simulink model "JointSpaceControl_own_MCP"  (R2013a)
settings: Solver=ode45  StartTime=0.0  StopTime=sim_end  MaxStep=0.008  RelTol=1e-3
PreLoadFcn:
  | Initialization
InitFcn:
  | Initialization
values from neighbouring files (symbols this model uses):
  a_max = [27 27 27 27 27 27]    [Initialization.m]
  dq_0 = qd_actual.signals.values(1,:)    [Initialization.m]
  K_0 = [            omega_1, zeros(1,5);         0,          omega_2, zeros(1,4);         zeros(1,2), omega_3, zeros(1,3);         zeros(1,3), omega_4, zeros(1,2);         zeros(1,4), omega_5, 0;         zeros(1,5), omega_6]    [Initialization.m]
  K_1 = [            omega_7, zeros(1,5);         0,          omega_8, zeros(1,4);         zeros(1,2), omega_9, zeros(1,3);         zeros(1,3), omega_10, zeros(1,2);         zeros(1,4), omega_11, 0;         zeros(1,5), omega_12]    [Initialization.m]
  q_0 = q_actual.signals.values(1,:)    [Initialization.m]
  q_max = 2*pi*ones(1,6)    [Initialization.m]
  q_min = -2*pi*ones(1,6)    [Initialization.m]
  torque_max = [150 150 150 28 28 28]    [Initialization.m]
  v_max = 3.4*ones(1,6)    [Initialization.m]
(part 3 of 4)

== matlab function JointSpaceControl_own_MCP/Forward & Velocity Kinematics Joint -> Tool Geometric Jacobian/J (made by Michael) ==
  data: J0 output; q input; Tn output
function [J0, Tn] = ur5_jacobian( q )
%UNTITLED J0 returns the jacobian in the inertial frame. Tn returns the
%transformation from origin to end-effector (forward kinematics).

%Defining input ports
q1 = q(1);
q2 = q(2);
q3 = q(3);
q4 = q(4);
q5 = q(5);
q6 = q(6);

% Jacobian (end-effector frame)
Jn1 = [ (35967658190210792782316868215998932771611847913227196662655717226173663198915229*cos(q5 - q6))/106799351796045504119751085308477605730135226117832638497352080391110986289032027501148104346828800 + (84451879200365687*sin(q2 - q6))/6490371073168534535663120411525120 + (194949711497644156173*sin(q4 - q6))/16225927682921336339157801028812800000 - (194949711497644156173*sin(q2 + q3 + q6))/16225927682921336339157801028812800000 + (275840770609662734656058457562955*sin(q2 + q5 + q6))/2596148429267413814265248164610048 - (84451879200365687*sin(q3 + q4 + q6))/6490371073168534535663120411525120 - (2053060087794098037004962814352767697732810782616901170279221510647830364092218317*sin(q4 + q5 + q6))/341757925747345613183203472987128338336432723577064443191526657251555156124902488003673933909852160 - (127350816012176408189502377060506389*sin(q2 + q3 - q5 - q6))/1298074214633706907132624082305024000 - (111172761678833366316347747967194492076366052381217435623730136019215778584537765*sin(q3 + q4 - q5 - q6))/17087896287367280659160173649356416916821636178853222159576332862577757806245124400183696695492608 + (519875567647652786170952659526825091883968323036151981961339556365617307809635277352352397416158688535123641112322663680196253259*cos(q2 + q3 + q4 + q5 - q6))/17329185588255092872365088650894273146477731721098853594815497378841383173785160143999840038150872363108695068508772323931088486400 + (2122825234561248616893610494268290878536612480468246686583653420460184422081415019027164128055730209555068108774478778867800150153*cos(q2 + q3 + q4 - q5 + q6))/86645927941275464361825443254471365732388658605494267974077486894206915868925800719999200190754361815543475342543861619655442432000 + (194949711497644156173*sin(q2 + q3 - q6))/16225927682921336339157801028812800000 + (1379203853048313504376533887083401*sin(q2 + q5 - q6))/12980742146337069071326240823050240 - (1379203853048313504376533887083401*sin(q2 - q5 + q6))/12980742146337069071326240823050240 + (84451879200365687*sin(q3 + q4 - q6))/6490371073168534535663120411525120 - (51326502194852444639440407923254275912386270512895480308024020327083350576388417787*sin(q4 + q5 - q6))/8543948143683640329580086824678208458410818089426611079788166431288878903122562200091848347746304000 - (1283162554871310958843918637192253228892250922824946721836627660932782523731312344957*sin(q4 - q5 + q6))/213598703592091008239502170616955211460270452235665276994704160782221972578064055002296208693657600000 + (191*cos(q2 + q3 + q4 + q6))/2000 + (127350816012176408189502377060506389*sin(q2 + q3 + q5 + q6))/1298074214633706907132624082305024000 - (111172761678833379931084422202676435483582369162931350478896764012094883767702875*sin(q3 + q4 + q5 + q6))/17087896287367280659160173649356416916821636178853222159576332862577757806245124400183696695492608 + (2861063719675858867154458072038785344359566180156884446265273330888120000481209071*cos(q5 + q6))/533996758980227520598755426542388028650676130589163192486760401955554931445160137505740521734144000 - (84451879200365687*sin(q2 + q6))/6490371073168534535663120411525120 - (194949711497644156173*sin(q4 + q6))/16225927682921336339157801028812800000 - (1429657811031045161970119813698793047136231009974723550987905358752535048856873346718200821789284381747153397866676246912996806793*cos(q2 + q3 + q4 - q5 - q6))/86645927941275464361825443254471365732388658605494267974077486894206915868925800719999200190754361815543475342543861619655442432000 - (1011823238475430797566174171647961*cos(q6))/3291009114642412084309938365114701009965471731267159726697218048000 - (275840770609662734656058457562955*sin(q2 - q5 - q6))/2596148429267413814265248164610048 - (51326502194852444639440407923254275912386270512895480308024020327083350576388417787*sin(q4 - q5 - q6))/8543948143683640329580086824678208458410818089426611079788166431288878903122562200091848347746304000 - (27*cos(q2 + q3 + q4 - q6))/2000 + (3183770400304409814838136431224347379*sin(q2 + q3 + q5 - q6))/32451855365842672678315602057625600000 - (3183770400304409814838136431224347379*sin(q2 + q3 - q5 + q6))/32451855365842672678315602057625600000 - (111172761678833366316347747967194492076366052381217435623730136019215778584537765*sin(q3 + q4 + q5 - q6))/17087896287367280659160173649356416916821636178853222159576332862577757806245124400183696695492608 - (555863808394166763508055368658571079967593346278931128385257758985228012726659783*sin(q3 + q4 - q5 + q6))/85439481436836403295800868246782084584108180894266110797881664312888789031225622000918483477463040 + (6151860883830558723075280489357521634050976598849036133515047236737481169606567320141085730345932291258072846594526784421861331081*cos(q2 + q3 + q4 + q5 + q6))/86645927941275464361825443254471365732388658605494267974077486894206915868925800719999200190754361815543475342543861619655442432000, (3772528186279210902532250340080927*cos(q5)*cos(q6))/40564819207303340847894502572032000 - (203678061600881951*cos(q6))/40564819207303340847894502572032000 - (39243*cos(q4)*sin(q6))/100000 - (269862747400677809654420514623322019689666659727888053949852700633*sin(q5)*sin(q6))/3291009114642412084309938365114701009965471731267159726697218048000 + (17*sin(q3)*sin(q4)*sin(q6))/40 + (194949711497644156173*sin(q4)*sin(q5)*sin(q6))/8112963841460668169578900514406400000 - (17*cos(q3)*cos(q4)*sin(q6))/40 - (968462910914422702168033488243437403*cos(q4)*cos(q5)*sin(q6))/658201822928482416861987673022940201993094346253431945339443609600000 - (194949711497644156173*cos(q4)*cos(q6)*sin(q5))/8112963841460668169578900514406400000 - (39243*cos(q5)*cos(q6)*sin(q4))/100000 - (419536464733715208746950266293057*cos(q3)*cos(q4)*cos(q5)*sin(q6))/263280729171392966744795069209176080797237738501372778135777443840 - (84451879200365687*cos(q3)*cos(q4)*cos(q6)*sin(q5))/3245185536584267267831560205762560 - (17*cos(q3)*cos(q5)*cos(q6)*sin(q4))/40 - (17*cos(q4)*cos(q5)*cos(q6)*sin(q3))/40 + (84451879200365687*cos(q3)*sin(q4)*sin(q5)*sin(q6))/3245185536584267267831560205762560 + (84451879200365687*cos(q4)*sin(q3)*sin(q5)*sin(q6))/3245185536584267267831560205762560 + (419536464733715208746950266293057*cos(q5)*sin(q3)*sin(q4)*sin(q6))/263280729171392966744795069209176080797237738501372778135777443840 + (84451879200365687*cos(q6)*sin(q3)*sin(q4)*sin(q5))/3245185536584267267831560205762560, (3772528186279210902532250340080927*cos(q5)*cos(q6))/40564819207303340847894502572032000 - (203678061600881951*cos(q6))/40564819207303340847894502572032000 - (39243*cos(q4)*sin(q6))/100000 - (269862747400677809654420514623322019689666659727888053949852700633*sin(q5)*sin(q6))/3291009114642412084309938365114701009965471731267159726697218048000 + (194949711497644156173*sin(q4)*sin(q5)*sin(q6))/8112963841460668169578900514406400000 - (968462910914422702168033488243437403*cos(q4)*cos(q5)*sin(q6))/658201822928482416861987673022940201993094346253431945339443609600000 - (194949711497644156173*cos(q4)*cos(q6)*sin(q5))/8112963841460668169578900514406400000 - (39243*cos(q5)*cos(q6)*sin(q4))/100000, (3772528186279210902532250340080927*cos(q5)*cos(q6))/40564819207303340847894502572032000 - (203678061600881951*cos(q6))/40564819207303340847894502572032000 - (269862747400677809654420514623322019689666659727888053949852700633*sin(q5)*sin(q6))/3291009114642412084309938365114701009965471731267159726697218048000,                                 -(41*cos(q6))/500, 0];
Jn2 = [ (35967658190210792782316868215998932771611847913227196662655717226173663198915229*sin(q5 - q6))/106799351796045504119751085308477605730135226117832638497352080391110986289032027501148104346828800 - (194949711497644156173*cos(q4 - q6))/16225927682921336339157801028812800000 - (6151860883830558723075280489357521634050976598849036133515047236737481169606567320141085730345932291258072846594526784421861331081*sin(q2 + q3 + q4 + q5 + q6))/86645927941275464361825443254471365732388658605494267974077486894206915868925800719999200190754361815543475342543861619655442432000 - (84451879200365687*cos(q2 - q6))/6490371073168534535663120411525120 - (194949711497644156173*cos(q2 + q3 + q6))/16225927682921336339157801028812800000 + (275840770609662734656058457562955*cos(q2 + q5 + q6))/2596148429267413814265248164610048 - (84451879200365687*cos(q3 + q4 + q6))/6490371073168534535663120411525120 - (2053060087794098037004962814352767697732810782616901170279221510647830364092218317*cos(q4 + q5 + q6))/341757925747345613183203472987128338336432723577064443191526657251555156124902488003673933909852160 + (127350816012176408189502377060506389*cos(q2 + q3 - q5 - q6))/1298074214633706907132624082305024000 + (111172761678833366316347747967194492076366052381217435623730136019215778584537765*cos(q3 + q4 - q5 - q6))/17087896287367280659160173649356416916821636178853222159576332862577757806245124400183696695492608 + (519875567647652786170952659526825091883968323036151981961339556365617307809635277352352397416158688535123641112322663680196253259*sin(q2 + q3 + q4 + q5 - q6))/17329185588255092872365088650894273146477731721098853594815497378841383173785160143999840038150872363108695068508772323931088486400 - (2122825234561248616893610494268290878536612480468246686583653420460184422081415019027164128055730209555068108774478778867800150153*sin(q2 + q3 + q4 - q5 + q6))/86645927941275464361825443254471365732388658605494267974077486894206915868925800719999200190754361815543475342543861619655442432000 - (194949711497644156173*cos(q2 + q3 - q6))/16225927682921336339157801028812800000 - (1379203853048313504376533887083401*cos(q2 + q5 - q6))/12980742146337069071326240823050240 - (1379203853048313504376533887083401*cos(q2 - q5 + q6))/12980742146337069071326240823050240 - (84451879200365687*cos(q3 + q4 - q6))/6490371073168534535663120411525120 + (51326502194852444639440407923254275912386270512895480308024020327083350576388417787*cos(q4 + q5 - q6))/8543948143683640329580086824678208458410818089426611079788166431288878903122562200091848347746304000 - (1283162554871310958843918637192253228892250922824946721836627660932782523731312344957*cos(q4 - q5 + q6))/213598703592091008239502170616955211460270452235665276994704160782221972578064055002296208693657600000 + (127350816012176408189502377060506389*cos(q2 + q3 + q5 + q6))/1298074214633706907132624082305024000 - (111172761678833379931084422202676435483582369162931350478896764012094883767702875*cos(q3 + q4 + q5 + q6))/17087896287367280659160173649356416916821636178853222159576332862577757806245124400183696695492608 - (191*sin(q2 + q3 + q4 + q6))/2000 - (84451879200365687*cos(q2 + q6))/6490371073168534535663120411525120 - (194949711497644156173*cos(q4 + q6))/16225927682921336339157801028812800000 - (2861063719675858867154458072038785344359566180156884446265273330888120000481209071*sin(q5 + q6))/533996758980227520598755426542388028650676130589163192486760401955554931445160137505740521734144000 - (1429657811031045161970119813698793047136231009974723550987905358752535048856873346718200821789284381747153397866676246912996806793*sin(q2 + q3 + q4 - q5 - q6))/86645927941275464361825443254471365732388658605494267974077486894206915868925800719999200190754361815543475342543861619655442432000 + (275840770609662734656058457562955*cos(q2 - q5 - q6))/2596148429267413814265248164610048 + (51326502194852444639440407923254275912386270512895480308024020327083350576388417787*cos(q4 - q5 - q6))/8543948143683640329580086824678208458410818089426611079788166431288878903122562200091848347746304000 + (1011823238475430797566174171647961*sin(q6))/3291009114642412084309938365114701009965471731267159726697218048000 - (3183770400304409814838136431224347379*cos(q2 + q3 + q5 - q6))/32451855365842672678315602057625600000 - (3183770400304409814838136431224347379*cos(q2 + q3 - q5 + q6))/32451855365842672678315602057625600000 + (111172761678833366316347747967194492076366052381217435623730136019215778584537765*cos(q3 + q4 + q5 - q6))/17087896287367280659160173649356416916821636178853222159576332862577757806245124400183696695492608 - (555863808394166763508055368658571079967593346278931128385257758985228012726659783*cos(q3 + q4 - q5 + q6))/85439481436836403295800868246782084584108180894266110797881664312888789031225622000918483477463040 - (27*sin(q2 + q3 + q4 - q6))/2000, (203678061600881951*sin(q6))/40564819207303340847894502572032000 - (39243*cos(q4)*cos(q6))/100000 - (3772528186279210902532250340080927*cos(q5)*sin(q6))/40564819207303340847894502572032000 - (269862747400677809654420514623322019689666659727888053949852700633*cos(q6)*sin(q5))/3291009114642412084309938365114701009965471731267159726697218048000 - (17*cos(q3)*cos(q4)*cos(q6))/40 - (968462910914422702168033488243437403*cos(q4)*cos(q5)*cos(q6))/658201822928482416861987673022940201993094346253431945339443609600000 + (17*cos(q6)*sin(q3)*sin(q4))/40 + (194949711497644156173*cos(q4)*sin(q5)*sin(q6))/8112963841460668169578900514406400000 + (39243*cos(q5)*sin(q4)*sin(q6))/100000 + (194949711497644156173*cos(q6)*sin(q4)*sin(q5))/8112963841460668169578900514406400000 - (419536464733715208746950266293057*cos(q3)*cos(q4)*cos(q5)*cos(q6))/263280729171392966744795069209176080797237738501372778135777443840 + (84451879200365687*cos(q3)*cos(q4)*sin(q5)*sin(q6))/3245185536584267267831560205762560 + (17*cos(q3)*cos(q5)*sin(q4)*sin(q6))/40 + (84451879200365687*cos(q3)*cos(q6)*sin(q4)*sin(q5))/3245185536584267267831560205762560 + (17*cos(q4)*cos(q5)*sin(q3)*sin(q6))/40 + (84451879200365687*cos(q4)*cos(q6)*sin(q3)*sin(q5))/3245185536584267267831560205762560 + (419536464733715208746950266293057*cos(q5)*cos(q6)*sin(q3)*sin(q4))/263280729171392966744795069209176080797237738501372778135777443840 - (84451879200365687*sin(q3)*sin(q4)*sin(q5)*sin(q6))/3245185536584267267831560205762560, (203678061600881951*sin(q6))/40564819207303340847894502572032000 - (39243*cos(q4)*cos(q6))/100000 - (3772528186279210902532250340080927*cos(q5)*sin(q6))/40564819207303340847894502572032000 - (269862747400677809654420514623322019689666659727888053949852700633*cos(q6)*sin(q5))/3291009114642412084309938365114701009965471731267159726697218048000 - (968462910914422702168033488243437403*cos(q4)*cos(q5)*cos(q6))/658201822928482416861987673022940201993094346253431945339443609600000 + (194949711497644156173*cos(q4)*sin(q5)*sin(q6))/8112963841460668169578900514406400000 + (39243*cos(q5)*sin(q4)*sin(q6))/100000 + (194949711497644156173*cos(q6)*sin(q4)*sin(q5))/8112963841460668169578900514406400000, (203678061600881951*sin(q6))/40564819207303340847894502572032000 - (3772528186279210902532250340080927*cos(q5)*sin(q6))/40564819207303340847894502572032000 - (269862747400677809654420514623322019689666659727888053949852700633*cos(q6)*sin(q5))/3291009114642412084309938365114701009965471731267159726697218048000,                                  (41*sin(q6))/500, 0];
Jn3 = [                                                                                                                                                                                                                                                                                                                                                                                                                                                                                                                                                                                                                                                                                                                                                                                                                                                                                                                                                                                                                                                                                                                                                                                                                                                                                                                                                                                                                                                                                                                                                                                                                                                                                                                                                                                                                                                                                                                                                                                                                                                                                                                                                                                                                                                                                                                                                                                                                                                                                                                                                                                                                                                                                                                                                                                                                                                                                                                                                                                                                                                                                                                                                                                                                                                                                                                               (17*cos(q2 - q5))/80 + (15816199602835760256257693185578612149839397336469669*cos(q4 - q5))/1316403645856964833723975346045880403986188692506863890678887219200000 + (39243*cos(q2 + q3 + q5))/200000 - (1370310084591942294341002243687833653188636725005*cos(q3 + q4 + q5))/105312291668557186697918027683670432318895095400549111254310977536 + (541485578402344699*sin(q2 + q3 + q4))/81129638414606681695789005144064000 + (39243*cos(q2 + q3 - q5))/200000 + (6851550422959710632632081751008750772042651038911*cos(q3 + q4 - q5))/526561458342785933489590138418352161594475477002745556271554887680 - (1329567682315534563473755419380555181845910000005711135641209403853*sin(q2 + q3 + q4 + q5))/13164036458569648337239753460458804039861886925068638906788872192000 + (968462910914422702168033488243437403*cos(q2 + q3))/658201822928482416861987673022940201993094346253431945339443609600000 + (17*cos(q2 + q5))/80 + (419536464733715208746950266293057*cos(q3 + q4))/263280729171392966744795069209176080797237738501372778135777443840 - (632647984113430487727340600576960659436254952933779*cos(q4 + q5))/52656145834278593348959013841835216159447547700274555627155488768000 + (419536464733715208746950266293057*cos(q2))/263280729171392966744795069209176080797237738501372778135777443840 + (968462910914422702168033488243437403*cos(q4))/658201822928482416861987673022940201993094346253431945339443609600000 - (462001456802000523*sin(q5))/81129638414606681695789005144064000 + (105312291668557180249399982545116558696073684159504065944814356019*sin(q2 + q3 + q4 - q5))/13164036458569648337239753460458804039861886925068638906788872192000,                                                                                                                                                                                                                                                                                                                                                                                                                                                                                                                                                                                                                                                                                                                                                                                                                                                                                                                                                                                       (3183770400304409814838136431224347379*cos(q4 - q5))/16225927682921336339157801028812800000 - (275840770609662734656058457562955*cos(q3 + q4 + q5))/1298074214633706907132624082305024 + (1379203853048313504376533887083401*cos(q3 + q4 - q5))/6490371073168534535663120411525120 + (84451879200365687*cos(q3 + q4))/3245185536584267267831560205762560 - (127350816012176408189502377060506389*cos(q4 + q5))/649037107316853453566312041152512000 + (194949711497644156173*cos(q4))/8112963841460668169578900514406400000 - (93*sin(q5))/1000,                                                                                                                                                                                                                                                                                                                                                                                                                                                                                                              (194949711497644156173*cos(q4))/8112963841460668169578900514406400000 - (93*sin(q5))/1000 - (194949711497644156173*cos(q4)*cos(q5))/8112963841460668169578900514406400000 + (39243*sin(q4)*sin(q5))/100000,                                                                                                                                                                                                                                                                                                     -(93*sin(q5))/1000,                                                 0, 0];
Jn4 = [                                                                                                                                                                                                                                                                                                                                                                                                                                                                                                                                                                                                                                                                                                                                                                                                                                                                                                                                                                                                                                                                                                                                                                                                                                                                                                                                                                                                                                                                                                                                                                                                                                                                                                                                                                                                                                                                                                                                                                                                                                                                                                                                                                                                                                                                                                                                                                                                                                                                                                                                                                                                                                                                                                                                                                                                                                                                                                                                                                                                                                                                                                                                                                                                                                                                                                                                                                                                                                                                                                                                                                                                                                                                                                                                                                                                                                                                                          (6582018229284824974684632372548374012493161295659483273165080625*sin(q2 + q3 + q4 + q5 + q6))/26328072917139296674479506920917608079723773850137277813577744384 + (403032377821159448978357750059338280708391237583*sin(q5 - q6))/13164036458569648337239753460458804039861886925068638906788872192 + (6582018229284824168619876730229377341315370891051451985731712975*sin(q2 + q3 + q4 + q5 - q6))/26328072917139296674479506920917608079723773850137277813577744384 + (6582018229284823362555121087910479384599870772374890568949237809*sin(q2 + q3 + q4 - q5 + q6))/26328072917139296674479506920917608079723773850137277813577744384 + sin(q2 + q3 + q4 + q6)/2 + (403032377821159498335588895202304015643716683825*sin(q5 + q6))/13164036458569648337239753460458804039861886925068638906788872192 + (6582018229284824168619876730229377341315370891051451985731712975*sin(q2 + q3 + q4 - q5 - q6))/26328072917139296674479506920917608079723773850137277813577744384 - (24678615572571482867467662723121*sin(q6))/6582018229284824168619876730229402019930943462534319453394436096 - sin(q2 + q3 + q4 - q6)/2,                                                                                                                                                                                                                                                                                                                                                                                                                                                                                                                                                                                                                                                                                                                                                                                                                                                                                                                                                                                                                                                                                                                                                                                                                                                                                                                                                                                                                             sin(q5) - (4967757600021511*sin(q5/2)^2*sin(q6))/40564819207303340847894502572032 - 2*sin(q6/2)^2*sin(q5),                                                                                                                                                                                                                                                                                                                                                                                                                                                                                                                                                                                                               sin(q5) - (4967757600021511*sin(q5/2)^2*sin(q6))/40564819207303340847894502572032 - 2*sin(q6/2)^2*sin(q5),                                                                                                                                                                                                              sin(q5) - (4967757600021511*sin(q5/2)^2*sin(q6))/40564819207303340847894502572032 - 2*sin(q6/2)^2*sin(q5),                                          -sin(q6), 0];
Jn5 = [                                                                                                                                                                                                                                                                                                                                                                                                                                                                                                                                                                                                                                                                                                                                                                                                                                                                                                                                                                                                                                                                                                                                                                                                                                                                                                                                                                                                                                                                                                                                                                                                                                                                                                                                                                                                                                                                                                                                                                                                                                                                                                                                                                                                                                                                                                                                                                                                                                                                                                                                                                                                                                                                                                                                                                                                                                                                                                                                                                                                                                                                                                                                                                                                                                                                                                                                                                                                                                                                                                                                                                                                                                                                                                                                                                                                                                                                                          (6582018229284823362555121087910479384599870772374890568949237809*cos(q2 + q3 + q4 - q5 + q6))/26328072917139296674479506920917608079723773850137277813577744384 - (6582018229284824168619876730229377341315370891051451985731712975*cos(q2 + q3 + q4 + q5 - q6))/26328072917139296674479506920917608079723773850137277813577744384 - (403032377821159448978357750059338280708391237583*cos(q5 - q6))/13164036458569648337239753460458804039861886925068638906788872192 + cos(q2 + q3 + q4 + q6)/2 + (403032377821159498335588895202304015643716683825*cos(q5 + q6))/13164036458569648337239753460458804039861886925068638906788872192 - (6582018229284824168619876730229377341315370891051451985731712975*cos(q2 + q3 + q4 - q5 - q6))/26328072917139296674479506920917608079723773850137277813577744384 - (24678615572571482867467662723121*cos(q6))/6582018229284824168619876730229402019930943462534319453394436096 + cos(q2 + q3 + q4 - q6)/2 + (6582018229284824974684632372548374012493161295659483273165080625*cos(q2 + q3 + q4 + q5 + q6))/26328072917139296674479506920917608079723773850137277813577744384,                                                                                                                                                                                                                                                                                                                                                                                                                                                                                                                                                                                                                                                                                                                                                                                                                                                                                                                                                                                                                                                                                                                                                                                                                                                                                                                                                                                   (4967757600021511*cos(q5)*cos(q6))/81129638414606681695789005144064 - (4967757600021511*cos(q6))/81129638414606681695789005144064 - sin(q5)*sin(q6),                                                                                                                                                                                                                                                                                                                                                                                                                                                                                                                                                                     (4967757600021511*cos(q5)*cos(q6))/81129638414606681695789005144064 - (4967757600021511*cos(q6))/81129638414606681695789005144064 - sin(q5)*sin(q6),                                                                                                                                                                    (4967757600021511*cos(q5)*cos(q6))/81129638414606681695789005144064 - (4967757600021511*cos(q6))/81129638414606681695789005144064 - sin(q5)*sin(q6),                                          -cos(q6), 0];
Jn6 = [                                                                                                                                                                                                                                                                                                                                                                                                                                                                                                                                                                                                                                                                                                                                                                                                                                                                                                                                                                                                                                                                                                                                                                                                                                                                                                                                                                                                                                                                                                                                                                                                                                                                                                                                                                                                                                                                                                                                                                                                                                                                                                                                                                                                                                                                                                                                                                                                                                                                                                                                                                                                                                                                                                                                                                                                                                                                                                                                                                                                                                                                                                                                                                                                                                                                                                                                                                                                                                                                                                                                                                                                                                                                                                                                                                                                                                                                                                                                                                                                                                                                                                                                                                                                                                                                                                                                                                                                                                                                                                                            (81129638414606686663546605165575*cos(q2 + q3 + q4 + q5))/162259276829213363391578010288128 - (4967757600021511*cos(q2 + q3 + q4))/81129638414606681695789005144064 + (4967757600021511*cos(q5))/81129638414606681695789005144064 - (81129638414606676728031405122553*cos(q2 + q3 + q4 - q5))/162259276829213363391578010288128 + 122597380068651197257713859414983140362437055831/533996758980227520598755426542388028650676130589163192486760401955554931445160137505740521734144,                                                                                                                                                                                                                                                                                                                                                                                                                                                                                                                                                                                                                                                                                                                                                                                                                                                                                                                                                                                                                                                                                                                                                                                                                                                                                                                                                                                                                           cos(q5) + 24678615572571482867467662723121/6582018229284824168619876730229402019930943462534319453394436096,                                                                                                                                                                                                                                                                                                                                                                                                                                                                                                                                                                                                             cos(q5) + 24678615572571482867467662723121/6582018229284824168619876730229402019930943462534319453394436096,                                                                                                                                                                                                            cos(q5) + 24678615572571482867467662723121/6582018229284824168619876730229402019930943462534319453394436096, 4967757600021511/81129638414606681695789005144064, 1];

% Forward kinematics
Tn1 = [   cos(q6)*(sin(q5)*(sin(q1) - (4967757600021511*cos(q4)*(sin(q3)*(cos(q1)*cos(q2) - (4967757600021511*sin(q1)*sin(q2))/81129638414606681695789005144064) + cos(q3)*(cos(q1)*sin(q2) + (4967757600021511*cos(q2)*sin(q1))/81129638414606681695789005144064)))/81129638414606681695789005144064 + (4967757600021511*sin(q4)*(sin(q3)*(cos(q1)*sin(q2) + (4967757600021511*cos(q2)*sin(q1))/81129638414606681695789005144064) - cos(q3)*(cos(q1)*cos(q2) - (4967757600021511*sin(q1)*sin(q2))/81129638414606681695789005144064)))/81129638414606681695789005144064) - cos(q5)*(cos(q4)*(sin(q3)*(cos(q1)*sin(q2) + (4967757600021511*cos(q2)*sin(q1))/81129638414606681695789005144064) - cos(q3)*(cos(q1)*cos(q2) - (4967757600021511*sin(q1)*sin(q2))/81129638414606681695789005144064)) + sin(q4)*(sin(q3)*(cos(q1)*cos(q2) - (4967757600021511*sin(q1)*sin(q2))/81129638414606681695789005144064) + cos(q3)*(cos(q1)*sin(q2) + (4967757600021511*cos(q2)*sin(q1))/81129638414606681695789005144064)))) + sin(q6)*((4967757600021511*cos(q5)*(sin(q1) - (4967757600021511*cos(q4)*(sin(q3)*(cos(q1)*cos(q2) - (4967757600021511*sin(q1)*sin(q2))/81129638414606681695789005144064) + cos(q3)*(cos(q1)*sin(q2) + (4967757600021511*cos(q2)*sin(q1))/81129638414606681695789005144064)))/81129638414606681695789005144064 + (4967757600021511*sin(q4)*(sin(q3)*(cos(q1)*sin(q2) + (4967757600021511*cos(q2)*sin(q1))/81129638414606681695789005144064) - cos(q3)*(cos(q1)*cos(q2) - (4967757600021511*sin(q1)*sin(q2))/81129638414606681695789005144064)))/81129638414606681695789005144064))/81129638414606681695789005144064 - (4967757600021511*sin(q1))/81129638414606681695789005144064 - cos(q4)*(sin(q3)*(cos(q1)*cos(q2) - (4967757600021511*sin(q1)*sin(q2))/81129638414606681695789005144064) + cos(q3)*(cos(q1)*sin(q2) + (4967757600021511*cos(q2)*sin(q1))/81129638414606681695789005144064)) + sin(q4)*(sin(q3)*(cos(q1)*sin(q2) + (4967757600021511*cos(q2)*sin(q1))/81129638414606681695789005144064) - cos(q3)*(cos(q1)*cos(q2) - (4967757600021511*sin(q1)*sin(q2))/81129638414606681695789005144064)) + (4967757600021511*sin(q5)*(cos(q4)*(sin(q3)*(cos(q1)*sin(q2) + (4967757600021511*cos(q2)*sin(q1))/81129638414606681695789005144064) - cos(q3)*(cos(q1)*cos(q2) - (4967757600021511*sin(q1)*sin(q2))/81129638414606681695789005144064)) + sin(q4)*(sin(q3)*(cos(q1)*cos(q2) - (4967757600021511*sin(q1)*sin(q2))/81129638414606681695789005144064) + cos(q3)*(cos(q1)*sin(q2) + (4967757600021511*cos(q2)*sin(q1))/81129638414606681695789005144064))))/81129638414606681695789005144064), cos(q6)*((4967757600021511*cos(q5)*(sin(q1) - (4967757600021511*cos(q4)*(sin(q3)*(cos(q1)*cos(q2) - (4967757600021511*sin(q1)*sin(q2))/81129638414606681695789005144064) + cos(q3)*(cos(q1)*sin(q2) + (4967757600021511*cos(q2)*sin(q1))/81129638414606681695789005144064)))/81129638414606681695789005144064 + (4967757600021511*sin(q4)*(sin(q3)*(cos(q1)*sin(q2) + (4967757600021511*cos(q2)*sin(q1))/81129638414606681695789005144064) - cos(q3)*(cos(q1)*cos(q2) - (4967757600021511*sin(q1)*sin(q2))/81129638414606681695789005144064)))/81129638414606681695789005144064))/81129638414606681695789005144064 - (4967757600021511*sin(q1))/81129638414606681695789005144064 - cos(q4)*(sin(q3)*(cos(q1)*cos(q2) - (4967757600021511*sin(q1)*sin(q2))/81129638414606681695789005144064) + cos(q3)*(cos(q1)*sin(q2) + (4967757600021511*cos(q2)*sin(q1))/81129638414606681695789005144064)) + sin(q4)*(sin(q3)*(cos(q1)*sin(q2) + (4967757600021511*cos(q2)*sin(q1))/81129638414606681695789005144064) - cos(q3)*(cos(q1)*cos(q2) - (4967757600021511*sin(q1)*sin(q2))/81129638414606681695789005144064)) + (4967757600021511*sin(q5)*(cos(q4)*(sin(q3)*(cos(q1)*sin(q2) + (4967757600021511*cos(q2)*sin(q1))/81129638414606681695789005144064) - cos(q3)*(cos(q1)*cos(q2) - (4967757600021511*sin(q1)*sin(q2))/81129638414606681695789005144064)) + sin(q4)*(sin(q3)*(cos(q1)*cos(q2) - (4967757600021511*sin(q1)*sin(q2))/81129638414606681695789005144064) + cos(q3)*(cos(q1)*sin(q2) + (4967757600021511*cos(q2)*sin(q1))/81129638414606681695789005144064))))/81129638414606681695789005144064) - sin(q6)*(sin(q5)*(sin(q1) - (4967757600021511*cos(q4)*(sin(q3)*(cos(q1)*cos(q2) - (4967757600021511*sin(q1)*sin(q2))/81129638414606681695789005144064) + cos(q3)*(cos(q1)*sin(q2) + (4967757600021511*cos(q2)*sin(q1))/81129638414606681695789005144064)))/81129638414606681695789005144064 + (4967757600021511*sin(q4)*(sin(q3)*(cos(q1)*sin(q2) + (4967757600021511*cos(q2)*sin(q1))/81129638414606681695789005144064) - cos(q3)*(cos(q1)*cos(q2) - (4967757600021511*sin(q1)*sin(q2))/81129638414606681695789005144064)))/81129638414606681695789005144064) - cos(q5)*(cos(q4)*(sin(q3)*(cos(q1)*sin(q2) + (4967757600021511*cos(q2)*sin(q1))/81129638414606681695789005144064) - cos(q3)*(cos(q1)*cos(q2) - (4967757600021511*sin(q1)*sin(q2))/81129638414606681695789005144064)) + sin(q4)*(sin(q3)*(cos(q1)*cos(q2) - (4967757600021511*sin(q1)*sin(q2))/81129638414606681695789005144064) + cos(q3)*(cos(q1)*sin(q2) + (4967757600021511*cos(q2)*sin(q1))/81129638414606681695789005144064)))), sin(q1 - q5)/2 - (6582018229284824974684632372548374012493161295659483273165080625*sin(q1 + q2 + q3 + q4 + q5))/26328072917139296674479506920917608079723773850137277813577744384 - (6582018229284823362555121087910479384599870772374890568949237809*sin(q1 - q2 - q3 - q4 + q5))/26328072917139296674479506920917608079723773850137277813577744384 + (6582018229284824168619876730229377341315370891051451985731712975*sin(q1 + q2 + q3 + q4 - q5))/26328072917139296674479506920917608079723773850137277813577744384 + (6582018229284824168619876730229377341315370891051451985731712975*sin(q1 - q2 - q3 - q4 - q5))/26328072917139296674479506920917608079723773850137277813577744384 + (403032377821159498335588895202304015643716683825*sin(q1 + q2 + q3 + q4))/13164036458569648337239753460458804039861886925068638906788872192 + sin(q1 + q5)/2 - (403032377821159448978357750059338280708391237583*sin(q1 - q2 - q3 - q4))/13164036458569648337239753460458804039861886925068638906788872192 + (24678615572571482867467662723121*sin(q1))/6582018229284824168619876730229402019930943462534319453394436096, (41*sin(q1 - q5))/1000 - (2158901979205422591696559418195866676097756904976310513598146445*sin(q1 + q2 + q3 + q4 + q5))/105312291668557186697918027683670432318895095400549111254310977536 - (1379203853048313504376533887083401*cos(q1 - q2))/6490371073168534535663120411525120 - (127350816012176408189502377060506389*cos(q1 + q2 + q3))/649037107316853453566312041152512000 - (269862747400677757864759964604329654768594701667370513326918750169*sin(q1 - q2 - q3 - q4 + q5))/13164036458569648337239753460458804039861886925068638906788872192000 + (10794509896027111636536597837576178839757208261324381256600009279*sin(q1 + q2 + q3 + q4 - q5))/526561458342785933489590138418352161594475477002745556271554887680 + (10794509896027111636536597837576178839757208261324381256600009279*sin(q1 - q2 - q3 - q4 - q5))/526561458342785933489590138418352161594475477002745556271554887680 + (12242553906469774364246293092284886029407723065419755446469379521*sin(q1 + q2 + q3 + q4))/263280729171392966744795069209176080797237738501372778135777443840 - (275840770609662734656058457562955*cos(q1 + q2))/1298074214633706907132624082305024 + (41*sin(q1 + q5))/1000 - (306063847661744321624146189939289076990197121107531973440372846631*sin(q1 - q2 - q3 - q4))/6582018229284824168619876730229402019930943462534319453394436096000 - (3183770400304409814838136431224347379*cos(q1 - q2 - q3))/16225927682921336339157801028812800000 + (358719993496022935930788850481418946958734396472101366570677587929*sin(q1))/3291009114642412084309938365114701009965471731267159726697218048000];
Tn2 = [ - cos(q6)*(sin(q5)*(cos(q1) + (4967757600021511*cos(q4)*(sin(q3)*((4967757600021511*cos(q1)*sin(q2))/81129638414606681695789005144064 + cos(q2)*sin(q1)) - cos(q3)*((4967757600021511*cos(q1)*cos(q2))/81129638414606681695789005144064 - sin(q1)*sin(q2))))/81129638414606681695789005144064 + (4967757600021511*sin(q4)*(sin(q3)*((4967757600021511*cos(q1)*cos(q2))/81129638414606681695789005144064 - sin(q1)*sin(q2)) + cos(q3)*((4967757600021511*cos(q1)*sin(q2))/81129638414606681695789005144064 + cos(q2)*sin(q1))))/81129638414606681695789005144064) - cos(q5)*(cos(q4)*(sin(q3)*((4967757600021511*cos(q1)*cos(q2))/81129638414606681695789005144064 - sin(q1)*sin(q2)) + cos(q3)*((4967757600021511*cos(q1)*sin(q2))/81129638414606681695789005144064 + cos(q2)*sin(q1))) - sin(q4)*(sin(q3)*((4967757600021511*cos(q1)*sin(q2))/81129638414606681695789005144064 + cos(q2)*sin(q1)) - cos(q3)*((4967757600021511*cos(q1)*cos(q2))/81129638414606681695789005144064 - sin(q1)*sin(q2))))) - sin(q6)*((4967757600021511*cos(q5)*(cos(q1) + (4967757600021511*cos(q4)*(sin(q3)*((4967757600021511*cos(q1)*sin(q2))/81129638414606681695789005144064 + cos(q2)*sin(q1)) - cos(q3)*((4967757600021511*cos(q1)*cos(q2))/81129638414606681695789005144064 - sin(q1)*sin(q2))))/81129638414606681695789005144064 + (4967757600021511*sin(q4)*(sin(q3)*((4967757600021511*cos(q1)*cos(q2))/81129638414606681695789005144064 - sin(q1)*sin(q2)) + cos(q3)*((4967757600021511*cos(q1)*sin(q2))/81129638414606681695789005144064 + cos(q2)*sin(q1))))/81129638414606681695789005144064))/81129638414606681695789005144064 - (4967757600021511*cos(q1))/81129638414606681695789005144064 + cos(q4)*(sin(q3)*((4967757600021511*cos(q1)*sin(q2))/81129638414606681695789005144064 + cos(q2)*sin(q1)) - cos(q3)*((4967757600021511*cos(q1)*cos(q2))/81129638414606681695789005144064 - sin(q1)*sin(q2))) + sin(q4)*(sin(q3)*((4967757600021511*cos(q1)*cos(q2))/81129638414606681695789005144064 - sin(q1)*sin(q2)) + cos(q3)*((4967757600021511*cos(q1)*sin(q2))/81129638414606681695789005144064 + cos(q2)*sin(q1))) + (4967757600021511*sin(q5)*(cos(q4)*(sin(q3)*((4967757600021511*cos(q1)*cos(q2))/81129638414606681695789005144064 - sin(q1)*sin(q2)) + cos(q3)*((4967757600021511*cos(q1)*sin(q2))/81129638414606681695789005144064 + cos(q2)*sin(q1))) - sin(q4)*(sin(q3)*((4967757600021511*cos(q1)*sin(q2))/81129638414606681695789005144064 + cos(q2)*sin(q1)) - cos(q3)*((4967757600021511*cos(q1)*cos(q2))/81129638414606681695789005144064 - sin(q1)*sin(q2)))))/81129638414606681695789005144064), sin(q6)*(sin(q5)*(cos(q1) + (4967757600021511*cos(q4)*(sin(q3)*((4967757600021511*cos(q1)*sin(q2))/81129638414606681695789005144064 + cos(q2)*sin(q1)) - cos(q3)*((4967757600021511*cos(q1)*cos(q2))/81129638414606681695789005144064 - sin(q1)*sin(q2))))/81129638414606681695789005144064 + (4967757600021511*sin(q4)*(sin(q3)*((4967757600021511*cos(q1)*cos(q2))/81129638414606681695789005144064 - sin(q1)*sin(q2)) + cos(q3)*((4967757600021511*cos(q1)*sin(q2))/81129638414606681695789005144064 + cos(q2)*sin(q1))))/81129638414606681695789005144064) - cos(q5)*(cos(q4)*(sin(q3)*((4967757600021511*cos(q1)*cos(q2))/81129638414606681695789005144064 - sin(q1)*sin(q2)) + cos(q3)*((4967757600021511*cos(q1)*sin(q2))/81129638414606681695789005144064 + cos(q2)*sin(q1))) - sin(q4)*(sin(q3)*((4967757600021511*cos(q1)*sin(q2))/81129638414606681695789005144064 + cos(q2)*sin(q1)) - cos(q3)*((4967757600021511*cos(q1)*cos(q2))/81129638414606681695789005144064 - sin(q1)*sin(q2))))) - cos(q6)*((4967757600021511*cos(q5)*(cos(q1) + (4967757600021511*cos(q4)*(sin(q3)*((4967757600021511*cos(q1)*sin(q2))/81129638414606681695789005144064 + cos(q2)*sin(q1)) - cos(q3)*((4967757600021511*cos(q1)*cos(q2))/81129638414606681695789005144064 - sin(q1)*sin(q2))))/81129638414606681695789005144064 + (4967757600021511*sin(q4)*(sin(q3)*((4967757600021511*cos(q1)*cos(q2))/81129638414606681695789005144064 - sin(q1)*sin(q2)) + cos(q3)*((4967757600021511*cos(q1)*sin(q2))/81129638414606681695789005144064 + cos(q2)*sin(q1))))/81129638414606681695789005144064))/81129638414606681695789005144064 - (4967757600021511*cos(q1))/81129638414606681695789005144064 + cos(q4)*(sin(q3)*((4967757600021511*cos(q1)*sin(q2))/81129638414606681695789005144064 + cos(q2)*sin(q1)) - cos(q3)*((4967757600021511*cos(q1)*cos(q2))/81129638414606681695789005144064 - sin(q1)*sin(q2))) + sin(q4)*(sin(q3)*((4967757600021511*cos(q1)*cos(q2))/81129638414606681695789005144064 - sin(q1)*sin(q2)) + cos(q3)*((4967757600021511*cos(q1)*sin(q2))/81129638414606681695789005144064 + cos(q2)*sin(q1))) + (4967757600021511*sin(q5)*(cos(q4)*(sin(q3)*((4967757600021511*cos(q1)*cos(q2))/81129638414606681695789005144064 - sin(q1)*sin(q2)) + cos(q3)*((4967757600021511*cos(q1)*sin(q2))/81129638414606681695789005144064 + cos(q2)*sin(q1))) - sin(q4)*(sin(q3)*((4967757600021511*cos(q1)*sin(q2))/81129638414606681695789005144064 + cos(q2)*sin(q1)) - cos(q3)*((4967757600021511*cos(q1)*cos(q2))/81129638414606681695789005144064 - sin(q1)*sin(q2)))))/81129638414606681695789005144064), (6582018229284823362555121087910479384599870772374890568949237809*cos(q1 - q2 - q3 - q4 + q5))/26328072917139296674479506920917608079723773850137277813577744384 - cos(q1 - q5)/2 - (6582018229284824168619876730229377341315370891051451985731712975*cos(q1 + q2 + q3 + q4 - q5))/26328072917139296674479506920917608079723773850137277813577744384 - (6582018229284824168619876730229377341315370891051451985731712975*cos(q1 - q2 - q3 - q4 - q5))/26328072917139296674479506920917608079723773850137277813577744384 - (403032377821159498335588895202304015643716683825*cos(q1 + q2 + q3 + q4))/13164036458569648337239753460458804039861886925068638906788872192 - cos(q1 + q5)/2 + (403032377821159448978357750059338280708391237583*cos(q1 - q2 - q3 - q4))/13164036458569648337239753460458804039861886925068638906788872192 - (24678615572571482867467662723121*cos(q1))/6582018229284824168619876730229402019930943462534319453394436096 + (6582018229284824974684632372548374012493161295659483273165080625*cos(q1 + q2 + q3 + q4 + q5))/26328072917139296674479506920917608079723773850137277813577744384, (269862747400677757864759964604329654768594701667370513326918750169*cos(q1 - q2 - q3 - q4 + q5))/13164036458569648337239753460458804039861886925068638906788872192000 - (1379203853048313504376533887083401*sin(q1 - q2))/6490371073168534535663120411525120 - (41*cos(q1 - q5))/1000 - (127350816012176408189502377060506389*sin(q1 + q2 + q3))/649037107316853453566312041152512000 - (10794509896027111636536597837576178839757208261324381256600009279*cos(q1 + q2 + q3 + q4 - q5))/526561458342785933489590138418352161594475477002745556271554887680 - (10794509896027111636536597837576178839757208261324381256600009279*cos(q1 - q2 - q3 - q4 - q5))/526561458342785933489590138418352161594475477002745556271554887680 - (12242553906469774364246293092284886029407723065419755446469379521*cos(q1 + q2 + q3 + q4))/263280729171392966744795069209176080797237738501372778135777443840 - (41*cos(q1 + q5))/1000 + (306063847661744321624146189939289076990197121107531973440372846631*cos(q1 - q2 - q3 - q4))/6582018229284824168619876730229402019930943462534319453394436096000 - (275840770609662734656058457562955*sin(q1 + q2))/1298074214633706907132624082305024 - (358719993496022935930788850481418946958734396472101366570677587929*cos(q1))/3291009114642412084309938365114701009965471731267159726697218048000 - (3183770400304409814838136431224347379*sin(q1 - q2 - q3))/16225927682921336339157801028812800000 + (2158901979205422591696559418195866676097756904976310513598146445*cos(q1 + q2 + q3 + q4 + q5))/105312291668557186697918027683670432318895095400549111254310977536];
Tn3 = [                                                                                                                                                                                                                                                                                                                                                                                                                                                                                                                                                                                                                                                                                                                                                                                                                                                                                                                                                                                                                                                                                                                                                                                                                                                                                                                                                                                                                                                                                                                                                                                                                                                                                                                                                                                                                                                                                                                                                                                 sin(q6)*(cos(q2 + q3 + q4) - (4967757600021511*sin(q2 + q3 + q4)*sin(q5))/81129638414606681695789005144064 + cos(q5)*((24678615572571482867467662723121*cos(q2 + q3 + q4))/6582018229284824168619876730229402019930943462534319453394436096 + 24678615572571482867467662723121/6582018229284824168619876730229402019930943462534319453394436096) - 24678615572571482867467662723121/6582018229284824168619876730229402019930943462534319453394436096) + cos(q6)*(sin(q2 + q3 + q4)*cos(q5) + sin(q5)*((4967757600021511*cos(q2 + q3 + q4))/81129638414606681695789005144064 + 4967757600021511/81129638414606681695789005144064)),                                                                                                                                                                                                                                                                                                                                                                                                                                                                                                                                                                                                                                                                                                                                                                                                                                                                                                                                                                                                                                                                                                                                                                                                                                                                                                                                                                                                                                                                                                                                                                                                                                                                                                                                                                                                                                                                                                                                                                               cos(q6)*(cos(q2 + q3 + q4) - (4967757600021511*sin(q2 + q3 + q4)*sin(q5))/81129638414606681695789005144064 + cos(q5)*((24678615572571482867467662723121*cos(q2 + q3 + q4))/6582018229284824168619876730229402019930943462534319453394436096 + 24678615572571482867467662723121/6582018229284824168619876730229402019930943462534319453394436096) - 24678615572571482867467662723121/6582018229284824168619876730229402019930943462534319453394436096) - sin(q6)*(sin(q2 + q3 + q4)*cos(q5) + sin(q5)*((4967757600021511*cos(q2 + q3 + q4))/81129638414606681695789005144064 + 4967757600021511/81129638414606681695789005144064)),                                                                                                                                                                                                                                                                                                                                                                                                                                                                                                                                                                                                                                                                                                                                           (4967757600021511*sin(q5/2)^2*sin(q2/2 + q3/2 + q4/2)^2)/20282409603651670423947251286016 - (4967757600021511*sin(q5/2)^2)/20282409603651670423947251286016 - sin(q2 + q3 + q4)*sin(q5) + 32697871082009813622455219990351566393691329179223172964110046442520659751916887/533996758980227520598755426542388028650676130589163192486760401955554931445160137505740521734144,                                                                                                                                                                                                                                                                                                                                                                                                                                                                                                                                                                                                                                                                                                                                                                                                                                                                                                                                                                                                                                                                 cos(q5)*((203678061600881951*cos(q2 + q3 + q4))/40564819207303340847894502572032000 + 203678061600881951/40564819207303340847894502572032000) - (39243*sin(q2 + q3))/100000 - (17*sin(q2))/40 - (3772528186279210902532250340080927*cos(q2 + q3 + q4))/40564819207303340847894502572032000 - (41*sin(q2 + q3 + q4)*sin(q5))/500 + 119081277252590746003692329966627208012012453867082549429325006754709186484175196065079416316417707/1334991897450568801496888566355970071626690326472907981216901004888887328612900343764351304335360000];
Tn4 = [                                                                                                                                                                                                                                                                                                                                                                                                                                                                                                                                                                                                                                                                                                                                                                                                                                                                                                                                                                                                                                                                                                                                                                                                                                                                                                                                                                                                                                                                                                                                                                                                                                                                                                                                                                                                                                                                                                                                                                                                                                                                                                                                                                                                                                                                                                                                                                                                                                                                                                                                                                                                                 0,                                                                                                                                                                                                                                                                                                                                                                                                                                                                                                                                                                                                                                                                                                                                                                                                                                                                                                                                                                                                                                                                                                                                                                                                                                                                                                                                                                                                                                                                                                                                                                                                                                                                                                                                                                                                                                                                                                                                                                                                                                                                                                                                                                                                                                                                                                                                                                                                                                                                                                                                                                                                               0,                                                                                                                                                                                                                                                                                                                                                                                                                                                                                                                                                                                                                                                                                                                                                                                                                                                                                                                                                                                                                                                                                                                     0,                                                                                                                                                                                                                                                                                                                                                                                                                                                                                                                                                                                                                                                                                                                                                                                                                                                                                                                                                                                                                                                                                                                                                                                                                                                                                                                                                                                                                                                                                                                                                                                                          1];


Jn = [Jn1; Jn2; Jn3; Jn4; Jn5; Jn6];
Tn = [Tn1; Tn2; Tn3; Tn4];
R = Tn(1:3,1:3);

% Jacobian (inertial frame)
J0 = [R, zeros(3,3); zeros(3,3), R] * Jn;


end
